simulink model "hw1"  (R2023a)
settings: Solver=ode4  StartTime=0.0  StopTime=2*86400  FixedStep=6  RelTol=1e-3
undefined symbols (not defined in the file or in its folder): plant
settings Model: Creator=ndelurgio  LastModifiedBy=ndelurgio

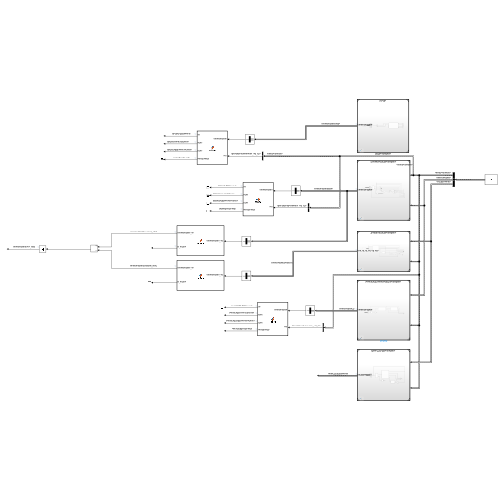
[thumbnail: Simulink's stored preview of the top-level diagram]
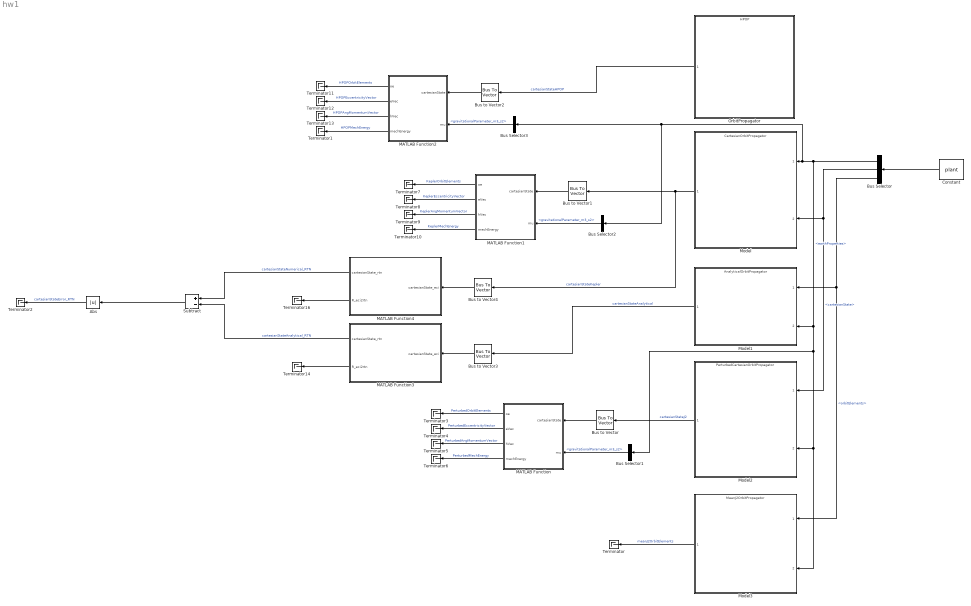
== system hw1 ==
  Abs : Abs  SaturateOnIntegerOverflow=off
  Bus Selector : BusSelector  OutputSignals=environment.earthProperties,chief.initialConditions.cartesianState,chief.initialConditions.orbitElements
  Bus Selector1 : BusSelector  OutputSignals=gravitationalParameter_m3_s2
  Bus Selector2 : BusSelector  OutputSignals=gravitationalParameter_m3_s2
  Bus Selector3 : BusSelector  OutputSignals=gravitationalParameter_m3_s2
  Bus to Vector{,1..4} (5 alike) : BusToVector
  Constant : Constant  Value=plant  OutDataTypeStr=Bus: plantBus
  MATLAB Function : MATLAB Function  TreatAsAtomicUnit=on
  MATLAB Function1 : MATLAB Function  TreatAsAtomicUnit=on
  MATLAB Function2 : MATLAB Function  TreatAsAtomicUnit=on
  MATLAB Function3 : MATLAB Function  TreatAsAtomicUnit=on
  MATLAB Function4 : MATLAB Function  TreatAsAtomicUnit=on
  Model : ModelReference  ModelNameDialog=CartesianOrbitPropagator.slx  SimulationMode=Normal  ModelReferenceVersion=1.43
  Model1 : ModelReference  ModelNameDialog=AnalyticalOrbitPropagator.slx  SimulationMode=Normal  ModelReferenceVersion=1.20
  Model2 : ModelReference  ModelNameDialog=PerturbedCartesianOrbitPropagator.slx  SimulationMode=Normal  ModelReferenceVersion=1.10
  Model3 : ModelReference  ModelNameDialog=MeanJ2OrbitPropagator.slx  SimulationMode=Normal  ModelReferenceVersion=1.32
  OrbitPropagator : ModelReference  ModelNameDialog=HPOP.slx  SimulationMode=Normal  ModelReferenceVersion=1.15
  Subtract : Sum  Inputs=+-
  Terminator{,1..14,16} (16 alike) : Terminator
  wires:
  Constant/1 -> Bus Selector/1
  Bus Selector/2 -> Model2/1, Model/2  "<cartesianState>"
  Model/1 -> Bus to Vector4/1, Bus to Vector1/1  "cartesianStateKepler"
  Bus Selector/3 -> Model3/1, Model1/1  "<orbitElements>"
  Model1/1 -> Bus to Vector3/1  "cartesianStateAnalytical"
  Model2/1 -> Bus to Vector/1  "cartesianStateJ2"
  Bus to Vector/1 -> MATLAB Function/1(cartesianState)
  Bus Selector1/1 -> MATLAB Function/2(mu)  "<gravitationalParameter_m3_s2>"
  MATLAB Function/1(oe) -> Terminator3/1  "PerturbedOrbitElements"
  MATLAB Function/2(eVec) -> Terminator4/1  "PerturbedEccentricityVector"
  MATLAB Function/3(hVec) -> Terminator5/1  "PerturbedAngMomentumVector"
  MATLAB Function/4(mechEnergy) -> Terminator6/1  "PerturbedMechEnergy"
  MATLAB Function1/1(oe) -> Terminator7/1  "KeplerOrbitElements"
  MATLAB Function1/4(mechEnergy) -> Terminator10/1  "KeplerMechEnergy"
  MATLAB Function1/3(hVec) -> Terminator9/1  "KeplerAngMomentumVector"
  Bus to Vector1/1 -> MATLAB Function1/1(cartesianState)
  MATLAB Function1/2(eVec) -> Terminator8/1  "KeplerEccentricityVector"
  Bus Selector2/1 -> MATLAB Function1/2(mu)  "<gravitationalParameter_m3_s2>"
  OrbitPropagator/1 -> Bus to Vector2/1  "cartesianStateHPOP"
  MATLAB Function2/2(eVec) -> Terminator12/1  "HPOPEccentricityVector"
  MATLAB Function2/1(oe) -> Terminator11/1  "HPOPOrbitElements"
  Bus Selector/1 -> Bus Selector3/1, Bus Selector2/1, Model/1, Bus Selector1/1, Model2/2, Model3/2, Model1/2  "<earthProperties>"
  Bus to Vector2/1 -> MATLAB Function2/1(cartesianState)
  MATLAB Function2/3(hVec) -> Terminator13/1  "HPOPAngMomentumVector"
  Bus Selector3/1 -> MATLAB Function2/2(mu)  "<gravitationalParameter_m3_s2>"
  MATLAB Function2/4(mechEnergy) -> Terminator1/1  "HPOPMechEnergy"
  Model3/1 -> Terminator/1  "meanJ2OrbitElements"
  Bus to Vector3/1 -> MATLAB Function3/1(cartesianState_eci)
  MATLAB Function3/1(cartesianState_rtn) -> Subtract/2  "cartesianStateAnalytical_RTN"
  MATLAB Function3/2(R_eci2rtn) -> Terminator14/1
  Bus to Vector4/1 -> MATLAB Function4/1(cartesianState_eci)
  MATLAB Function4/1(cartesianState_rtn) -> Subtract/1  "cartesianStateNumerical_RTN"
  MATLAB Function4/2(R_eci2rtn) -> Terminator16/1
  Subtract/1 -> Abs/1
  Abs/1 -> Terminator2/1  "cartesianStateError_RTN"

== matlab function hw1/MATLAB Function1 ==
  data: cartesianState input; oe output; mu input; eVec output; hVec output; mechEnergy output
function [oe,eVec,hVec,mechEnergy] = eci2oe ( cartesianState , mu )

[oe,eVec,hVec,mechEnergy] = eci2oe ( cartesianState , mu );

end

== matlab function hw1/MATLAB Function ==
  data: cartesianState input; oe output; mu input; eVec output; hVec output; mechEnergy output
function [oe,eVec,hVec,mechEnergy] = eci2oe ( cartesianState , mu )

[oe,eVec,hVec,mechEnergy] = eci2oe ( cartesianState , mu );

end

== matlab function hw1/MATLAB Function2 ==
  data: cartesianState input; oe output; mu input; eVec output; hVec output; mechEnergy output
function [oe,eVec,hVec,mechEnergy] = eci2oe ( cartesianState , mu )

[oe,eVec,hVec,mechEnergy] = eci2oe ( cartesianState , mu );

end

== matlab function hw1/MATLAB Function3 ==
  data: cartesianState_eci input; cartesianState_rtn output; R_eci2rtn output
function [cartesianState_rtn, R_eci2rtn] = eci2rtn(cartesianState_eci)
[cartesianState_rtn, R_eci2rtn] = eci2rtn(cartesianState_eci);
end

== matlab function hw1/MATLAB Function4 ==
  data: cartesianState_eci input; cartesianState_rtn output; R_eci2rtn output
function [cartesianState_rtn, R_eci2rtn] = eci2rtn(cartesianState_eci)
[cartesianState_rtn, R_eci2rtn] = eci2rtn(cartesianState_eci);
end
